simulink model "GIT_Shared_Model_Example"  (R2019b)
settings: Solver=FixedStepDiscrete  StartTime=0.0  StopTime=10  FixedStep=0.01  RelTol=1e-3  EnableMultiTasking=on
InitFcn:
  | clear mex;
undefined symbols (not defined in the file): asbcbaseini_C, ibatini_C, k_icalpl_C, scsocini_C, stopengstmode_C, t_bmaxini_C, t_bminini_C, t_vminddstr_C, TSB_Coulomb_float, TSB_Dc_float, TSB_Pwr_float, TSB_R_float, TSB_Soc, TSB_Tbatt, TSB_Tbatt_float, TSB_value_float, TSB_Volt_float, v_bcini_C, v_bcmaxini_C
libraries: Utility_Block_Library x22, AMO_Block_Library x2
(part 1 of 5)
settings Model: Creator=j0714063  LastModifiedBy=mhanif
settings ConfigSet: Description=|
  | AMOの標準コンフィギュレーションセット
  | 
  | Rev0.1  / 2022.06.10 / A.Maruyama
  | FixedStepSizeを参照形式に変更
  | 
  | Rev0.0  / 2022.04.26 / H.Kojima
  | 新規作成
settings DataIOCC: LimitDataPoints=on  SaveFormat=StructureWithTime  ReturnWorkspaceOutputs=off
settings OptimizationCC: DefaultParameterBehavior=Inlined  GainParamInheritBuiltInType=on  UseFloatMulNetSlope=on  DefaultUnderspecifiedDataType=single  EnhancedBackFolding=on  PassReuseOutputArgsAs=Individual arguments  ExpressionDepthLimit=2147483647  ZeroExternalMemoryAtStartup=off  ZeroInternalMemoryAtStartup=off  OptimizeBlockOrder=speed  DifferentSizesBufferReuse=on  OptimizationCustomize=off  EfficientTunableParamExpr=on
settings DebuggingCC: SignalInfNanChecking=error  SignalRangeChecking=error  ReadBeforeWriteMsg=EnableAllAsError  WriteAfterWriteMsg=EnableAllAsError  WriteAfterReadMsg=EnableAllAsError  AlgebraicLoopMsg=error  ArtificialAlgebraicLoopMsg=error  SaveWithDisabledLinksMsg=none  SaveWithParameterizedLinksMsg=error  BlockPriorityViolationMsg=error  MinStepSizeMsg=error  TimeAdjustmentMsg=warning  SolverPrmCheckMsg=error  InheritedTsInSrcMsg=error  SingleTaskRateTransMsg=error  TasksWithSamePriorityMsg=error  SigSpecEnsureSampleTimeMsg=error  CheckMatrixSingularityMsg=error  ParameterUnderflowMsg=error  ParameterTunabilityLossMsg=error  FixptConstUnderflowMsg=warning  FixptConstOverflowMsg=warning  FixptConstPrecisionLossMsg=warning  UnderSpecifiedDataTypeMsg=error  UnnecessaryDatatypeConvMsg=warning  VectorMatrixConversionMsg=warning  UnconnectedInputMsg=error  UnconnectedOutputMsg=error  UnconnectedLineMsg=error  SFcnCompatibilityMsg=error  UniqueDataStoreMsg=error  BusObjectLabelMismatch=error  RootOutportRequireBusObject=error  AllowSymbolicDim=off  ModelReferenceIOMsg=error  ModelReferenceVersionMismatchMessage=error  ModelReferenceIOMismatchMessage=error  UnknownTsInhSupMsg=error  ModelReferenceDataLoggingMessage=error  StateNameClashWarn=warning  OperatingPointInterfaceChecksumMismatchMsg=error  StrictBusMsg=ErrorOnBusTreatedAsVector  BusNameAdapt=ErrorWithoutRepair  NonBusSignalsTreatedAsBus=error  SFUnusedDataAndEventsDiag=error  SFInvalidInputDataAccessInChartInitDiag=error  SFTransitionOutsideNaturalParentDiag=error  SFUnreachableExecutionPathDiag=error  SFUndirectedBroadcastEventsDiag=error  SFTransitionActionBeforeConditionDiag=error  SFTemporalDelaySmallerThanSampleTimeDiag=error  SFSelfTransitionDiag=error  SFExecutionAtInitializationDiag=none  SFMachineParentedDataDiag=error  ForceCombineOutputUpdateInSim=on
settings HardwareCC: ProdBitPerPointer=32  ProdBitPerSizeT=32  ProdBitPerPtrDiffT=32  ProdLargestAtomicFloat=None  ProdWordSize=32  ProdHWDeviceType=Infineon->TriCore
settings ModelReferenceCC: ModelReferenceNumInstancesAllowed=Single  PropagateSignalLabelsOutOfModel=off
settings SFSimCC: SimUseLocalCustomCode=off  SimParseCustomCode=off  SimGenImportedTypeDefs=on  CompileTimeRecursionLimit=0  EnableRuntimeRecursion=off  MATLABDynamicMemAlloc=off  DefaultCustomCodeFunctionArrayLayout=Row-major  CustomCodeUndefinedFunction=UseInterfaceOnly
settings SFSimCC: SimCustomHeaderCode=|
  | #include "CommonFunction.h"
  | #include "def.h"
  | #include "float.h"
  | #include "hgsfloat.h"
  | #include "hos.h"
  | #include "kn_sfm.h"
  | #include "knos.h"
  | #include "Method.h"
  | #include "osdef.h"
  | #include "tl_basetypes.h"
  | #include "typedef.h"
  | #include "hgsub.h"
  | #include "hw.h"
  | #include "dsfxp.h"
  | #include "hv-plctrcvinfo10ms01-20p00-0.h"
  | #include "hv-plctrcvinfo10ms01-20p00-0_extdata.h"
  | #include "hv-plctrcvinfo10ms01-20p00-0_input.h"
settings SFSimCC: SimUserSources=|
  | ".\..\..\..\Utility\Helper_Modules\eagle\Add.c"
  | ".\..\..\..\Utility\Helper_Modules\eagle\CommonFunction.c"
  | ".\..\..\..\Utility\Helper_Modules\eagle\GE_Cal_fdivf.c"
  | ".\..\..\..\Utility\Helper_Modules\eagle\Ge_stdfunc2-osl-0.c"
  | ".\..\..\..\Utility\Helper_Modules\eagle\Ge_stdfuncmdl-os_-0.c"
  | ".\..\..\..\Utility\Helper_Modules\eagle\Ge_stdfunc-osl-0.c"
  | ".\..\..\..\Utility\Helper_Modules\eagle\Method.c"
  | ".\..\..\..\Utility\Helper_Modules\eagle\MulDiv.c"
  | ".\..\..\..\Utility\Helper_Modules\eagle\hgsub.c"
  | ".\..\..\..\Utility\Helper_Modules\eagle\GE_Lmt_f.c"
  | ".\..\..\..\Utility\Helper_Modules\eagle\J_get_PLCT.c"
  | ".\..\SRC\hv-plctrcvinfo10ms01-20p00-0.c"
  | ".\..\SRC\hv-plctrcvinfo10ms01-20p00-0_extdata.c"
  | ".\..\SRC\hv-plctrcvinfo10ms01-20p00-0_input.c"
settings SFSimCC: SimUserIncludeDirs=|
  | ".\..\..\..\Utility\Helper_Modules\eagle"
  | ".\..\SRC"
  | ".\..\..\..\Utility\Helper_Modules\TargetLink"
settings RTWCC: SystemTargetFile=ert.tlc  GenCodeOnly=on  TemplateMakefile=ert_default_tmf  GenerateReport=on  RTWUseLocalCustomCode=off  IncludeHyperlinkInReport=on  LaunchReport=on  GenerateTraceInfo=on  GenerateTraceReport=on  GenerateTraceReportSl=on  GenerateTraceReportSf=on  GenerateTraceReportEml=on  RTWCompilerOptimization=on
settings CodeAppCC: ForceParamTrailComments=on  IgnoreCustomStorageClasses=off  OperatorAnnotations=on  SimulinkDataObjDesc=on  SFDataObjDesc=on  InsertBlockDesc=on
settings ERTTargetCC: UtilityFuncGeneration=Shared location  GenerateSampleERTMain=on  SuppressErrorStatus=on  GenerateSharedConstants=off  InlinedParameterPlacement=NonHierarchical  ERTCustomFileTemplate=example_file_process.tlc  EnableDataOwnership=on
settings ConfigComp: CovMetricSettings=dcmtw  CovHtmlReporting=on  CovSaveCumulativeToWorkspaceVar=on  CovSaveSingleToWorkspaceVar=on  CovExternalEMLEnable=off

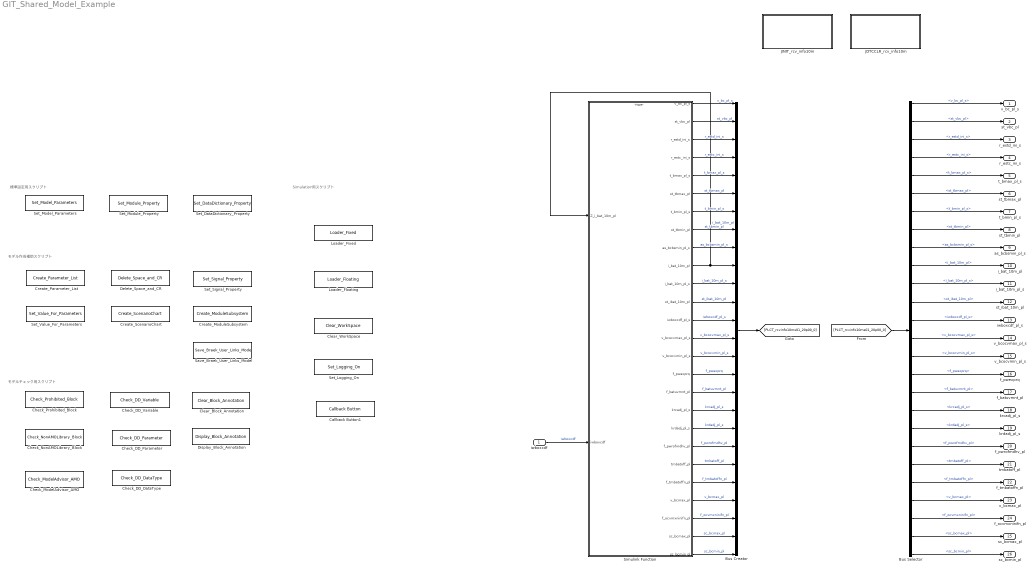
== system GIT_Shared_Model_Example ==
  note: 標準設定用スクリプト
  note: Simulation用スクリプト
  note: モデルチェック用スクリプト
  note: モデル作成補助スクリプト
  iwboxcdf : Inport  Tag=#AMO_Lib
      settings: AttributesFormatString=%<Tag>\n%<Description>\nSampleTime = %<SampleTime>
  Bus Creator : BusCreator  Inputs=26
  Bus Selector : BusSelector  OutputSignals=v_bc_pl_s,st_vbc_pl,r_estd_ini_s,r_estc_ini_s,t_bmax_pl_s,st_tbmax_pl,t_bmin_pl_s,st_tbmin_pl,as_bcbsmin_pl_s,i_bat_10m_pl,i_bat_10m_pl_s,st_ibat_10m_pl,iwboxcdf_pl_s,v_bcocvmax_pl_s,v_bcocvmin_pl_s,f_pwexprq,f_batuvmnt_pl,krcadj_pl_s,krdadj_pl_s,f_pwrofmdhv_pl,tmbatoff_pl,f_tmbatoffn_pl,v_bcmax_pl,f_ocvmxninifn_pl,sc_bcmax_pl,sc_bcmin_pl
  Callback Button1 : CallbackButton  Description=メモリの解放  ButtonText=Clear MEX
      settings: AttributesFormatString=%<Description>  ClickFcn=clear mex;
  Check_DD_DataType : Utility_Block_Library/Utility m-file Blocks/Check_DD_DataType  Description=|  SystemSampleTime=-1  Latency=0  AutoFrameSizeCalculation=off
      | DDのDataTypeと
      | モデル定義の整合性チェック
      settings: AttributesFormatString=%<Description>  SourceProductName=Utility_Block_Library
  Check_DD_Parameter : Utility_Block_Library/Utility m-file Blocks/Check_DD_Parameter  Description=|  SystemSampleTime=-1  Latency=0  AutoFrameSizeCalculation=off
      | 下記ブロックとDDの整合性チェック
      | Constant,Saturation,LookUpTable,Relay
      settings: AttributesFormatString=%<Description>  SourceProductName=Utility_Block_Library
  Check_DD_Variable : Utility_Block_Library/Utility m-file Blocks/Check_DD_Variable  Description=|  SystemSampleTime=-1  Latency=0  AutoFrameSizeCalculation=off
      | ポートブロック名、信号名とDDの整合性チェック
      | 強調表示の解除は　Ctrl+Shift+H
      settings: AttributesFormatString=%<Description>  SourceProductName=Utility_Block_Library
  Check_ModelAdvisor_AMO : Utility_Block_Library/Utility m-file Blocks/Check_ModelAdvisor_AMO  Description=|
      | AMO標準設定の状態で
      | ModelAdvisorを開く
      settings: AttributesFormatString=%<Description>  SourceProductName=Utility_Block_Library
  Check_NonAMOLibrary_Block : Utility_Block_Library/Utility m-file Blocks/Check_NonAMOLibrary_Block  Description=|
      | AMOライブラリー以外の
      | ブロックの有無をチェック
      settings: AttributesFormatString=%<Description>  SourceProductName=Utility_Block_Library
  Check_Prohibited_Block : Utility_Block_Library/Utility m-file Blocks/Check_Prohibited_Block  Description=AMOガイドラインで使用禁止とされている\nブロックの有無をチェック  SystemSampleTime=-1  Latency=0  AutoFrameSizeCalculation=off
      settings: AttributesFormatString=%<Description>  SourceProductName=Utility_Block_Library
  Clear_Block_Annotation : Utility_Block_Library/Utility m-file Blocks/Clear_Block_Annotation  Description=確認用に表示したブロックプロパティをクリア  SystemSampleTime=-1  Latency=0  AutoFrameSizeCalculation=off
      settings: AttributesFormatString=%<Description>  SourceProductName=Utility_Block_Library
  Clear_WorkSpace : Utility_Block_Library/Utility m-file Blocks/Clear_WorkSpace  SystemSampleTime=-1  Latency=0  AutoFrameSizeCalculation=off
      settings: AttributesFormatString=ワークスペースをクリア  SourceProductName=Utility_Block_Library
  Create_ModuleSubsystem : Utility_Block_Library/Utility m-file Blocks/Create_ModuleSubsystem  Description=DataDictionaryからBlankModuleを作成します  SystemSampleTime=-1  Latency=0  AutoFrameSizeCalculation=off
      settings: AttributesFormatString=%<Description>  SourceProductName=Utility_Block_Library
  Create_Parameter_List : Utility_Block_Library/Utility m-file Blocks/Create_Parameter_List  Description=モデル内で使われている変数リストを出力する  SystemSampleTime=-1  Latency=0  AutoFrameSizeCalculation=off
      settings: AttributesFormatString=%<Description>  SourceProductName=Utility_Block_Library
  Create_ScenarioChart : Utility_Block_Library/Utility m-file Blocks/Create_ScenarioChart  Description=シミュレーション用のシナリオチャート作成  SystemSampleTime=-1  Latency=0  AutoFrameSizeCalculation=off
      settings: AttributesFormatString=%<Description>  SourceProductName=Utility_Block_Library
  Delete_Space_and_CR : Utility_Block_Library/Utility m-file Blocks/Delete_Space_and_CR  Description=ポートブロック名から空白と改行を削除  SystemSampleTime=-1  Latency=0  AutoFrameSizeCalculation=off
      settings: AttributesFormatString=%<Description>  SourceProductName=Utility_Block_Library
  Display_Block_Annotation : Utility_Block_Library/Utility m-file Blocks/Display_Block_Annotation  Description=ブロックプロパティ確認用  SystemSampleTime=-1  Latency=0  AutoFrameSizeCalculation=off
      settings: AttributesFormatString=%<Description>  SourceProductName=Utility_Block_Library
  JDTCCLR_rcv_info10m : Subsystem  TreatAsAtomicUnit=on
  JINIT_rcv_info10m : Subsystem  TreatAsAtomicUnit=on
  Loader_Fixed : Utility_Block_Library/Utility m-file Blocks/Loader_Fixed  SystemSampleTime=-1  Latency=0  AutoFrameSizeCalculation=off
      settings: AttributesFormatString=固定小数点シミュレーションに必要なデータを\nワークスペースに展開  SourceProductName=Utility_Block_Library
  Loader_Floating : Utility_Block_Library/Utility m-file Blocks/Loader_Floating  SystemSampleTime=-1  Latency=0  AutoFrameSizeCalculation=off
      settings: AttributesFormatString=浮動小数点シミュレーションに必要なデータを\nワークスペースに展開  SourceProductName=Utility_Block_Library
  Save_Braek_User_Links_Model : Utility_Block_Library/Utility m-file Blocks/Save_Braek_User_Links_Model  Description=ユーザーライブラリへのリンクを切ったモデルを別名保存\n(ファイル名+BreakUserLinks.slxして保存)  SystemSampleTime=-1  Latency=0  AutoFrameSizeCalculation=off
      settings: AttributesFormatString=%<Description>  SourceProductName=Utility_Block_Library
  Set_DataDictionary_Property : Utility_Block_Library/Utility m-file Blocks/Set_DataDictionary_Property  Description=以下のスクリプトを実行します\nProperty_Port.m/ Property_Define.m / Property_Parameter.m\n[警告]\nモデルのポート名と同じ信号名を持つSignalBuilderブロックが存在するモデルで\n実行すると、SignalBuilderの内部プロパティが上書きされてしまい、\nシミュレーションエラーとなります  SystemSampleTime=-1  Latency=0  AutoFrameSizeCalculation=off
      settings: AttributesFormatString=%<Description>  SourceProductName=Utility_Block_Library
  Set_Logging_On : Utility_Block_Library/Utility m-file Blocks/Set_Logging_On  Description=名前の設定された信号をロギングする
      settings: AttributesFormatString=%<Description>  SourceProductName=Utility_Block_Library
  Set_Model_Parameters : Utility_Block_Library/Utility m-file Blocks/Set_Model_Parameters  Description=AMO標準のモデルプロパティ設定  SystemSampleTime=-1  Latency=0  AutoFrameSizeCalculation=off
      settings: AttributesFormatString=%<Description>  SourceProductName=Utility_Block_Library
  Set_Module_Property : Utility_Block_Library/Utility m-file Blocks/Set_Module_Property  Description=ModuleモデルサブシステムをAMO標準の\nスタイル及びAtomicに設定  SystemSampleTime=-1  Latency=0  AutoFrameSizeCalculation=off
      settings: AttributesFormatString=%<Description>  SourceProductName=Utility_Block_Library
  Set_Signal_Property : Utility_Block_Library/Utility m-file Blocks/Set_Signal_Property  Description=|  SystemSampleTime=-1  Latency=0  AutoFrameSizeCalculation=off
      | モジュールモデルサブシステムに対して
      | 信号名を作成＆オブジェクト関連付け
      settings: AttributesFormatString=%<Description>  SourceProductName=Utility_Block_Library
  Set_Value_For_Parameters : Utility_Block_Library/Utility m-file Blocks/Set_Value_For_Parameters  Description=Parameter定義されたブロックの値を設定  SystemSampleTime=-1  Latency=0  AutoFrameSizeCalculation=off
      settings: AttributesFormatString=%<Description>  SourceProductName=Utility_Block_Library
  Simulink Function : Subsystem  TreatAsAtomicUnit=on
  v_bc_pl_s : Outport  Tag=#AMO_Lib  SignalName=v_bc_pl_s
      settings: AttributesFormatString=%<Tag>\n%<Description>\nInitialOutput = %<InitialOutput>  MustResolveToSignalObject=on
  st_vbc_pl : Outport  Tag=#AMO_Lib  Port=2  SignalName=st_vbc_pl
      settings: AttributesFormatString=%<Tag>\n%<Description>\nInitialOutput = %<InitialOutput>  MustResolveToSignalObject=on
  r_estd_ini_s : Outport  Tag=#AMO_Lib  Port=3  SignalName=r_estd_ini_s
      settings: AttributesFormatString=%<Tag>\n%<Description>\nInitialOutput = %<InitialOutput>  MustResolveToSignalObject=on
  r_estc_ini_s : Outport  Tag=#AMO_Lib  Port=4  SignalName=r_estc_ini_s
      settings: AttributesFormatString=%<Tag>\n%<Description>\nInitialOutput = %<InitialOutput>  MustResolveToSignalObject=on
  t_bmax_pl_s : Outport  Tag=#AMO_Lib  Port=5  SignalName=t_bmax_pl_s
      settings: AttributesFormatString=%<Tag>\n%<Description>\nInitialOutput = %<InitialOutput>  MustResolveToSignalObject=on
  st_tbmax_pl : Outport  Tag=#AMO_Lib  Port=6  SignalName=st_tbmax_pl
      settings: AttributesFormatString=%<Tag>\n%<Description>\nInitialOutput = %<InitialOutput>  MustResolveToSignalObject=on
  t_bmin_pl_s : Outport  Tag=#AMO_Lib  Port=7  SignalName=t_bmin_pl_s
      settings: AttributesFormatString=%<Tag>\n%<Description>\nInitialOutput = %<InitialOutput>  MustResolveToSignalObject=on
  st_tbmin_pl : Outport  Tag=#AMO_Lib  Port=8  SignalName=st_tbmin_pl
      settings: AttributesFormatString=%<Tag>\n%<Description>\nInitialOutput = %<InitialOutput>  MustResolveToSignalObject=on
  as_bcbsmin_pl_s : Outport  Tag=#AMO_Lib  Port=9  SignalName=as_bcbsmin_pl_s
      settings: AttributesFormatString=%<Tag>\n%<Description>\nInitialOutput = %<InitialOutput>  MustResolveToSignalObject=on
  i_bat_10m_pl : Outport  Tag=#AMO_Lib  Port=10  SignalName=i_bat_10m_pl
      settings: AttributesFormatString=%<Tag>\n%<Description>\nInitialOutput = %<InitialOutput>  MustResolveToSignalObject=on
  i_bat_10m_pl_s : Outport  Tag=#AMO_Lib  Port=11  SignalName=i_bat_10m_pl_s
      settings: AttributesFormatString=%<Tag>\n%<Description>\nInitialOutput = %<InitialOutput>  MustResolveToSignalObject=on
  st_ibat_10m_pl : Outport  Tag=#AMO_Lib  Port=12  SignalName=st_ibat_10m_pl
      settings: AttributesFormatString=%<Tag>\n%<Description>\nInitialOutput = %<InitialOutput>  MustResolveToSignalObject=on
  iwboxcdf_pl_s : Outport  Tag=#AMO_Lib  Port=13  SignalName=iwboxcdf_pl_s
      settings: AttributesFormatString=%<Tag>\n%<Description>\nInitialOutput = %<InitialOutput>  MustResolveToSignalObject=on
  v_bcocvmax_pl_s : Outport  Tag=#AMO_Lib  Port=14  SignalName=v_bcocvmax_pl_s
      settings: AttributesFormatString=%<Tag>\n%<Description>\nInitialOutput = %<InitialOutput>  MustResolveToSignalObject=on
  v_bcocvmin_pl_s : Outport  Tag=#AMO_Lib  Port=15  SignalName=v_bcocvmin_pl_s
      settings: AttributesFormatString=%<Tag>\n%<Description>\nInitialOutput = %<InitialOutput>  MustResolveToSignalObject=on
  f_pwexprq : Outport  Tag=#AMO_Lib  Port=16  SignalName=f_pwexprq
      settings: AttributesFormatString=%<Tag>\n%<Description>\nInitialOutput = %<InitialOutput>  MustResolveToSignalObject=on
  f_batuvmnt_pl : Outport  Tag=#AMO_Lib  Port=17  SignalName=f_batuvmnt_pl
      settings: AttributesFormatString=%<Tag>\n%<Description>\nInitialOutput = %<InitialOutput>  MustResolveToSignalObject=on
  krcadj_pl_s : Outport  Tag=#AMO_Lib  Port=18  SignalName=krcadj_pl_s
      settings: AttributesFormatString=%<Tag>\n%<Description>\nInitialOutput = %<InitialOutput>  MustResolveToSignalObject=on
  krdadj_pl_s : Outport  Tag=#AMO_Lib  Port=19  SignalName=krdadj_pl_s
      settings: AttributesFormatString=%<Tag>\n%<Description>\nInitialOutput = %<InitialOutput>  MustResolveToSignalObject=on
  f_pwrofmdhv_pl : Outport  Tag=#AMO_Lib  Port=20  SignalName=f_pwrofmdhv_pl
      settings: AttributesFormatString=%<Tag>\n%<Description>\nInitialOutput = %<InitialOutput>  MustResolveToSignalObject=on
  tmbatoff_pl : Outport  Tag=#AMO_Lib  Port=21  SignalName=tmbatoff_pl
      settings: AttributesFormatString=%<Tag>\n%<Description>\nInitialOutput = %<InitialOutput>  MustResolveToSignalObject=on
  f_tmbatoffn_pl : Outport  Tag=#AMO_Lib  Port=22  SignalName=f_tmbatoffn_pl
      settings: AttributesFormatString=%<Tag>\n%<Description>\nInitialOutput = %<InitialOutput>  MustResolveToSignalObject=on
  v_bcmax_pl : Outport  Tag=#AMO_Lib  Port=23  SignalName=v_bcmax_pl
      settings: AttributesFormatString=%<Tag>\n%<Description>\nInitialOutput = %<InitialOutput>  MustResolveToSignalObject=on
  f_ocvmxninifn_pl : Outport  Tag=#AMO_Lib  Port=24  SignalName=f_ocvmxninifn_pl
      settings: AttributesFormatString=%<Tag>\n%<Description>\nInitialOutput = %<InitialOutput>  MustResolveToSignalObject=on
  sc_bcmax_pl : Outport  Tag=#AMO_Lib  Port=25  SignalName=sc_bcmax_pl
      settings: AttributesFormatString=%<Tag>\n%<Description>\nInitialOutput = %<InitialOutput>  MustResolveToSignalObject=on
  sc_bcmin_pl : Outport  Tag=#AMO_Lib  Port=26  SignalName=sc_bcmin_pl
      settings: AttributesFormatString=%<Tag>\n%<Description>\nInitialOutput = %<InitialOutput>  MustResolveToSignalObject=on
  wires:
  Bus Creator/1 -> [PLCT_rcvinfo10ms01_20p00_0]
  [PLCT_rcvinfo10ms01_20p00_0] -> Bus Selector/1
  Simulink Function/1(v_bc_pl_s) -> Bus Creator/1  "v_bc_pl_s"
  Simulink Function/2(st_vbc_pl) -> Bus Creator/2  "st_vbc_pl"
  Simulink Function/3(r_estd_ini_s) -> Bus Creator/3  "r_estd_ini_s"
  Simulink Function/4(r_estc_ini_s) -> Bus Creator/4  "r_estc_ini_s"
  Simulink Function/5(t_bmax_pl_s) -> Bus Creator/5  "t_bmax_pl_s"
  Simulink Function/6(st_tbmax_pl) -> Bus Creator/6  "st_tbmax_pl"
  Simulink Function/7(t_bmin_pl_s) -> Bus Creator/7  "t_bmin_pl_s"
  Simulink Function/8(st_tbmin_pl) -> Bus Creator/8  "st_tbmin_pl"
  Simulink Function/9(as_bcbsmin_pl_s) -> Bus Creator/9  "as_bcbsmin_pl_s"
  Simulink Function/10(i_bat_10m_pl) -> Simulink Function/1(Z_i_bat_10m_pl), Bus Creator/10  "i_bat_10m_pl"
  Simulink Function/11(i_bat_10m_pl_s) -> Bus Creator/11  "i_bat_10m_pl_s"
  Simulink Function/12(st_ibat_10m_pl) -> Bus Creator/12  "st_ibat_10m_pl"
  Simulink Function/13(iwboxcdf_pl_s) -> Bus Creator/13  "iwboxcdf_pl_s"
  Simulink Function/14(v_bcocvmax_pl_s) -> Bus Creator/14  "v_bcocvmax_pl_s"
  Simulink Function/15(v_bcocvmin_pl_s) -> Bus Creator/15  "v_bcocvmin_pl_s"
  Simulink Function/16(f_pwexprq) -> Bus Creator/16  "f_pwexprq"
  Simulink Function/17(f_batuvmnt_pl) -> Bus Creator/17  "f_batuvmnt_pl"
  Simulink Function/18(krcadj_pl_s) -> Bus Creator/18  "krcadj_pl_s"
  Simulink Function/19(krdadj_pl_s) -> Bus Creator/19  "krdadj_pl_s"
  Simulink Function/20(f_pwrofmdhv_pl) -> Bus Creator/20  "f_pwrofmdhv_pl"
  Simulink Function/21(tmbatoff_pl) -> Bus Creator/21  "tmbatoff_pl"
  Simulink Function/22(f_tmbatoffn_pl) -> Bus Creator/22  "f_tmbatoffn_pl"
  Simulink Function/23(v_bcmax_pl) -> Bus Creator/23  "v_bcmax_pl"
  Simulink Function/24(f_ocvmxninifn_pl) -> Bus Creator/24  "f_ocvmxninifn_pl"
  Simulink Function/25(sc_bcmax_pl) -> Bus Creator/25  "sc_bcmax_pl"
  Simulink Function/26(sc_bcmin_pl) -> Bus Creator/26  "sc_bcmin_pl"
  Bus Selector/1 -> v_bc_pl_s/1  "<v_bc_pl_s>"
  Bus Selector/2 -> st_vbc_pl/1  "<st_vbc_pl>"
  Bus Selector/3 -> r_estd_ini_s/1  "<r_estd_ini_s>"
  Bus Selector/4 -> r_estc_ini_s/1  "<r_estc_ini_s>"
  Bus Selector/5 -> t_bmax_pl_s/1  "<t_bmax_pl_s>"
  Bus Selector/6 -> st_tbmax_pl/1  "<st_tbmax_pl>"
  Bus Selector/7 -> t_bmin_pl_s/1  "<t_bmin_pl_s>"
  Bus Selector/8 -> st_tbmin_pl/1  "<st_tbmin_pl>"
  Bus Selector/9 -> as_bcbsmin_pl_s/1  "<as_bcbsmin_pl_s>"
  Bus Selector/10 -> i_bat_10m_pl/1  "<i_bat_10m_pl>"
  Bus Selector/11 -> i_bat_10m_pl_s/1  "<i_bat_10m_pl_s>"
  Bus Selector/12 -> st_ibat_10m_pl/1  "<st_ibat_10m_pl>"
  Bus Selector/13 -> iwboxcdf_pl_s/1  "<iwboxcdf_pl_s>"
  Bus Selector/14 -> v_bcocvmax_pl_s/1  "<v_bcocvmax_pl_s>"
  Bus Selector/15 -> v_bcocvmin_pl_s/1  "<v_bcocvmin_pl_s>"
  Bus Selector/16 -> f_pwexprq/1  "<f_pwexprq>"
  Bus Selector/17 -> f_batuvmnt_pl/1  "<f_batuvmnt_pl>"
  Bus Selector/18 -> krcadj_pl_s/1  "<krcadj_pl_s>"
  Bus Selector/19 -> krdadj_pl_s/1  "<krdadj_pl_s>"
  Bus Selector/20 -> f_pwrofmdhv_pl/1  "<f_pwrofmdhv_pl>"
  Bus Selector/21 -> tmbatoff_pl/1  "<tmbatoff_pl>"
  Bus Selector/22 -> f_tmbatoffn_pl/1  "<f_tmbatoffn_pl>"
  Bus Selector/23 -> v_bcmax_pl/1  "<v_bcmax_pl>"
  Bus Selector/24 -> f_ocvmxninifn_pl/1  "<f_ocvmxninifn_pl>"
  Bus Selector/25 -> sc_bcmax_pl/1  "<sc_bcmax_pl>"
  Bus Selector/26 -> sc_bcmin_pl/1  "<sc_bcmin_pl>"
  iwboxcdf/1 -> Simulink Function/2(iwboxcdf)  "iwboxcdf"
